simulink model "PosControl_Sim_PID"  (R2018a)
settings: Solver=ode4  StartTime=0.0  StopTime=8  FixedStep=0.001  RelTol=1e-3
InitFcn:
  | Init_control;
values from neighbouring files (symbols this model uses):
  CONSTANTS_ONE_G = 9.8    [Init_control.m]
  DEG2RAD = 0.0174533    [Init_control.m]
  FLT_EPSILON = 1e-5    (= 1e-05)    [Init_control.m]
  MAX_CONTROL_ANGLE_RATE_PITCH = 220    [Init_control.m]
  MAX_CONTROL_ANGLE_RATE_ROLL = 220    [Init_control.m]
  MAX_CONTROL_ANGLE_RATE_Y = 200    [Init_control.m]
  MAX_CONTROL_VELOCITY_XY = 5*2    (= 10)    [Init_control.m]
  MAX_CONTROL_VELOCITY_Z = 3*2    (= 6)    [Init_control.m]
  MC_PITCH_P = 6.5    [Init_control.m]
  MC_PITCHRATE_D = 0.0005    [Init_control.m]
  MC_PITCHRATE_I = 0.2    [Init_control.m]
  MC_PITCHRATE_P = 0.06    [Init_control.m]
  MC_ROLL_P = 11.5    [Init_control.m]
  MC_ROLLRATE_D = 0.0005    [Init_control.m]
  MC_ROLLRATE_I = 0.2    [Init_control.m]
  MC_ROLLRATE_P = 0.055    [Init_control.m]
  MC_YAW_P = 2.8    [Init_control.m]
  MC_YAW_WEIGHT = 0.4    [Init_control.m]
  MC_YAWRATE_D = 0.00    (= 0)    [Init_control.m]
  MC_YAWRATE_I = 0.1    [Init_control.m]
  MC_YAWRATE_P = 0.2    [Init_control.m]
  MPC_THR_MAX = 0.9    [Init_control.m]
  MPC_THR_MIN = 0.06    [Init_control.m]
  MPC_THR_XY_MARG = 0.3    [Init_control.m]
  MPC_TILTMAX_AIR = 90    [Init_control.m]
  MPC_XY_P = 2.2    [Init_control.m]
  MPC_XY_VEL_D_ACC = 0.2    [Init_control.m]
  MPC_XY_VEL_I_ACC = 0.4    [Init_control.m]
  MPC_XY_VEL_P_ACC = 4.0    (= 4)    [Init_control.m]
  MPC_Z_P = 0.8    [Init_control.m]
  MPC_Z_VEL_D_ACC = 0.0    (= 0)    [Init_control.m]
  MPC_Z_VEL_I_ACC = 2.0    (= 2)    [Init_control.m]
  MPC_Z_VEL_P_ACC = 4.0    (= 4)    [Init_control.m]
  Saturation_I_ah = 3.43    [Init_control.m]
  Saturation_I_az = 5    [Init_control.m]
  Saturation_I_RP_Max = 0.3    [Init_control.m]
  Saturation_I_RP_Min = -0.3    [Init_control.m]
  Saturation_I_Y_Max = 0.2    [Init_control.m]
  Saturation_I_Y_Min = -0.2    [Init_control.m]
  THR_HOVER = 0.331    [Init_control.m]
undefined symbols (not defined in the file or in its folder): DiscIntNeverNeededParam, earthRadius, ModelInit_AngEuler, ModelInit_PosE, ModelInit_Rads, ModelInit_RateB, ModelInit_VelB, ModelParam_envGravityAcc, ModelParam_motorCr, ModelParam_motorJm, ModelParam_motorT, ModelParam_motorWb, ModelParam_rotorCm, ModelParam_rotorCt, ModelParam_uavCCm, ModelParam_uavCd, ModelParam_uavJ, ModelParam_uavMass, ModelParam_uavR
libraries: simulink x7, sharedutil x2, aerolibfltsims x2, aerolibanimutils x1
(part 1 of 2)
settings Model: Creator=wsh  LastModifiedBy=truel
settings DebuggingCC: BusObjectLabelMismatch=error
settings CodeAppCC: StateflowObjectComments=on

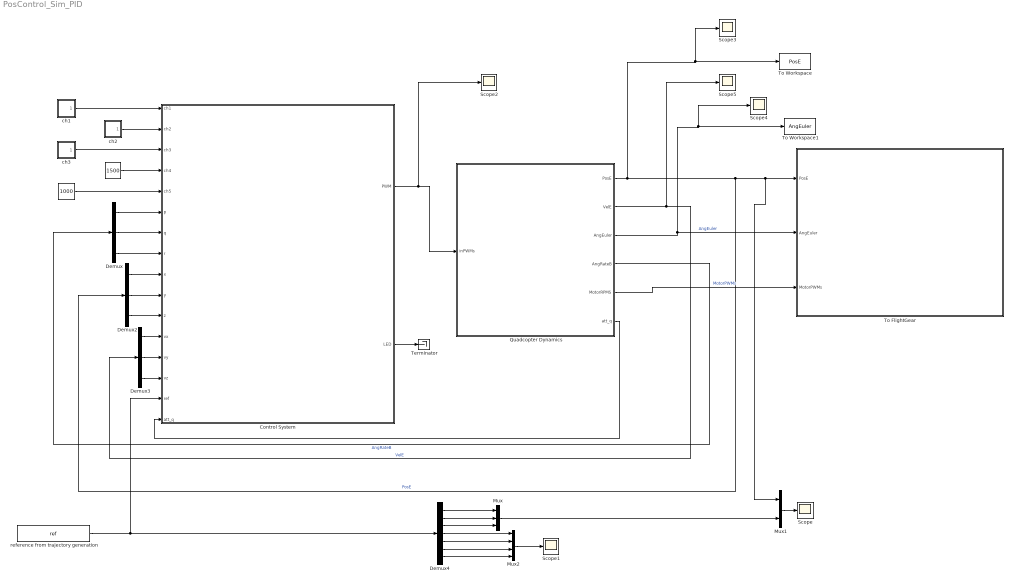
== system PosControl_Sim_PID ==
  " " : Constant  Value=1000  OutDataTypeStr=uint16
  "          " : Constant  Value=1500  OutDataTypeStr=uint16
  Control System : Subsystem
      mask Display: image('icon\pixhawk.png');
  Demux : Demux  Outputs=3
  Demux2 : Demux  Outputs=3
  Demux3 : Demux  Outputs=3
  Demux4 : Demux  Outputs=7
  Mux : Mux  Inputs=3
  Mux1 : Mux  Inputs=2
  Mux2 : Mux
  Quadcopter Dynamics : Subsystem
      mask Display: image('./icon/F450.png');
  Scope{,1..5} (6 alike) : Scope
  Terminator : Terminator
  To FlightGear : Subsystem
      mask Display: image('./icon/FlightGear.png');
  To Workspace : ToWorkspace  VariableName=PosE  SaveFormat=Structure With Time  SampleTime=-1
  To Workspace1 : ToWorkspace  VariableName=AngEuler  SaveFormat=Structure With Time  SampleTime=-1
  ch1 : Subsystem
  ch2 : Subsystem
  ch3 : Subsystem
  reference from trajectory generation : FromWorkspace  VariableName=ref  SampleTime=0
  wires:
  Quadcopter Dynamics/1(PosE) -> Demux2/1, Mux1/1, To FlightGear/1(PosE), To Workspace/1, Scope3/1  "PosE"
  Quadcopter Dynamics/5(MotorRPMS) -> To FlightGear/3(MotorPWMs)  "MotorPWMs"
  Control System/2(LED) -> Terminator/1
  Quadcopter Dynamics/3(AngEuler) -> To Workspace1/1, Scope4/1, To FlightGear/2(AngEuler)  "AngEuler"
  "          "/1 -> Control System/4(ch4)
  Quadcopter Dynamics/4(AngRateB) -> Demux/1  "AngRateB"
  " "/1 -> Control System/5(ch5)
  Demux/1 -> Control System/6(p)
  Demux/2 -> Control System/7(q)
  Demux/3 -> Control System/8(r)
  Demux2/1 -> Control System/9(x)
  Demux2/2 -> Control System/10(y)
  Demux2/3 -> Control System/11(z)
  Demux3/1 -> Control System/12(vx)
  Demux3/2 -> Control System/13(vy)
  Demux3/3 -> Control System/14(vz)
  Quadcopter Dynamics/2(VelE) -> Scope5/1, Demux3/1  "VelE"
  ch2/1(ch2) -> Control System/2(ch2)
  ch3/1(ch3) -> Control System/3(ch3)
  Control System/1(PWM) -> Scope2/1, Quadcopter Dynamics/1(inPWMs)
  reference from trajectory generation/1 -> Control System/15(ref), Demux4/1
  Demux4/1 -> Mux/1
  Demux4/2 -> Mux/2
  Demux4/3 -> Mux/3
  Mux1/1 -> Scope/1
  Mux/1 -> Mux1/2
  Demux4/4 -> Mux2/1
  Demux4/5 -> Mux2/2
  Demux4/6 -> Mux2/3
  Demux4/7 -> Mux2/4
  Mux2/1 -> Scope1/1
  Quadcopter Dynamics/6(att_q) -> Control System/16(att_q)
  ch1/1(ch1) -> Control System/1(ch1)

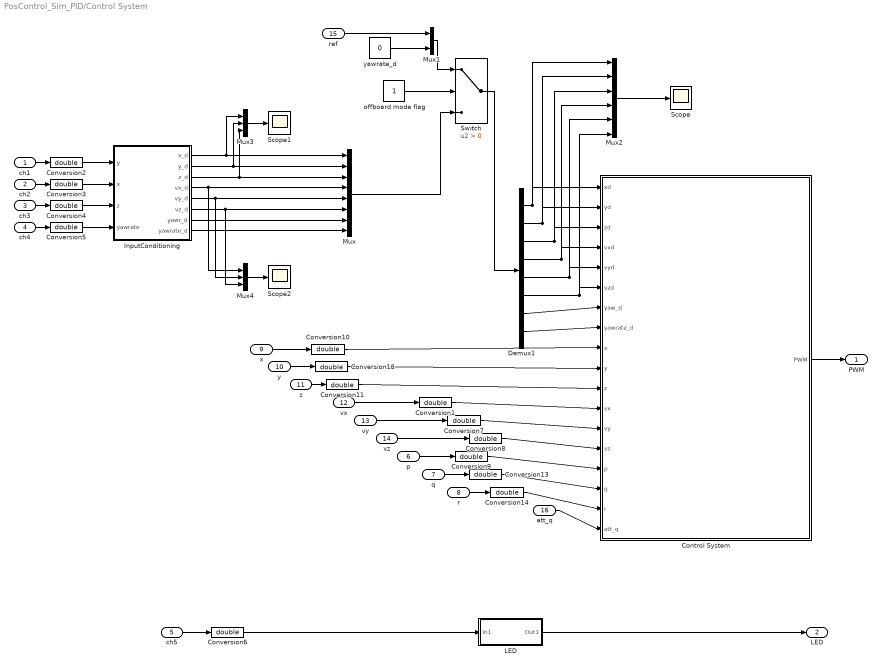
== system PosControl_Sim_PID/Control System ==
  ch1 : Inport  OutDataTypeStr=uint16  PortDimensions=1
  ch2 : Inport  Port=2  OutDataTypeStr=uint16  PortDimensions=1
  ch3 : Inport  Port=3  OutDataTypeStr=uint16  PortDimensions=1
  ch4 : Inport  Port=4  OutDataTypeStr=uint16  PortDimensions=1
  ch5 : Inport  Port=5  OutDataTypeStr=uint16  PortDimensions=1  Interpolate=off
  p : Inport  Port=6  PortDimensions=1
  q : Inport  Port=7  PortDimensions=1
  r : Inport  Port=8  PortDimensions=1
  x : Inport  Port=9
  y : Inport  Port=10
  z : Inport  Port=11
  vx : Inport  Port=12
  vy : Inport  Port=13
  vz : Inport  Port=14
  ref : Inport  Port=15
  att_q : Inport  Port=16  PortDimensions=[1 4]
  Control System : Subsystem
  Conversion{1..11,13..14,18} (14 alike) : DataTypeConversion  OutDataTypeStr=double
  Demux1 : Demux  Outputs=8
  InputConditioning : Subsystem
  "LED " : Subsystem
  Mux : Mux  Inputs=8
  Mux1 : Mux  Inputs=2
  Mux2 : Mux  Inputs=6
  Mux3 : Mux  Inputs=3
  Mux4 : Mux  Inputs=3
  Scope : Scope
  Scope1 : Scope
  Scope2 : Scope
  Switch : Switch  Criteria=u2 > Threshold
  offboard mode flag : Constant
  yawrate_d : Constant  Value=0
  PWM : Outport
  LED : Outport  Port=2  PortDimensions=1
  wires:
  ch3/1 -> Conversion4/1
  ch5/1 -> Conversion6/1
  ch4/1 -> Conversion5/1
  "LED "/1(Out1) -> LED/1
  Conversion6/1 -> "LED "/1(In1)
  Conversion5/1 -> InputConditioning/4("yawrate ")
  Control System/1(PWM) -> PWM/1
  ch1/1 -> Conversion2/1
  ch2/1 -> Conversion3/1
  y/1 -> Conversion18/1
  z/1 -> Conversion11/1
  vy/1 -> Conversion7/1
  Conversion10/1 -> Control System/9(x)
  Conversion18/1 -> Control System/10(y)
  Conversion11/1 -> Control System/11(z)
  Conversion2/1 -> InputConditioning/1(y)
  Conversion3/1 -> InputConditioning/2(x)
  vx/1 -> Conversion1/1
  Conversion1/1 -> Control System/12(vx)
  Conversion7/1 -> Control System/13(vy)
  vz/1 -> Conversion8/1
  Conversion8/1 -> Control System/14(vz)
  p/1 -> Conversion9/1
  q/1 -> Conversion13/1
  r/1 -> Conversion14/1
  Conversion9/1 -> Control System/15(p)
  Conversion13/1 -> Control System/16(q)
  Conversion14/1 -> Control System/17(r)
  Conversion4/1 -> InputConditioning/3(z)
  x/1 -> Conversion10/1
  offboard mode flag/1 -> Switch/2
  ref/1 -> Mux1/1
  yawrate_d/1 -> Mux1/2
  Mux1/1 -> Switch/1
  Mux/1 -> Switch/3
  Switch/1 -> Demux1/1
  Demux1/1 -> Control System/1(xd), Mux2/1
  Demux1/3 -> Control System/3(zd), Mux2/3
  Demux1/4 -> Mux2/4, Control System/4(vxd)
  Demux1/5 -> Mux2/5, Control System/5(vyd)
  Demux1/6 -> Mux2/6, Control System/6(vzd)
  Demux1/8 -> Control System/8(yawrate_d)
  Demux1/7 -> Control System/7(yaw_d)
  att_q/1 -> Control System/18(att_q)
  Mux2/1 -> Scope/1
  Demux1/2 -> Control System/2(yd), Mux2/2
  Mux3/1 -> Scope1/1
  InputConditioning/1(x_d) -> Mux3/1, Mux/1
  InputConditioning/2(y_d) -> Mux3/2, Mux/2
  InputConditioning/3(z_d) -> Mux3/3, Mux/3
  InputConditioning/7(yawr_d) -> Mux/7
  InputConditioning/8(yawrate_d) -> Mux/8
  Mux4/1 -> Scope2/1
  InputConditioning/4(vx_d) -> Mux4/1, Mux/4
  InputConditioning/5(vy_d) -> Mux4/2, Mux/5
  InputConditioning/6(vz_d) -> Mux4/3, Mux/6

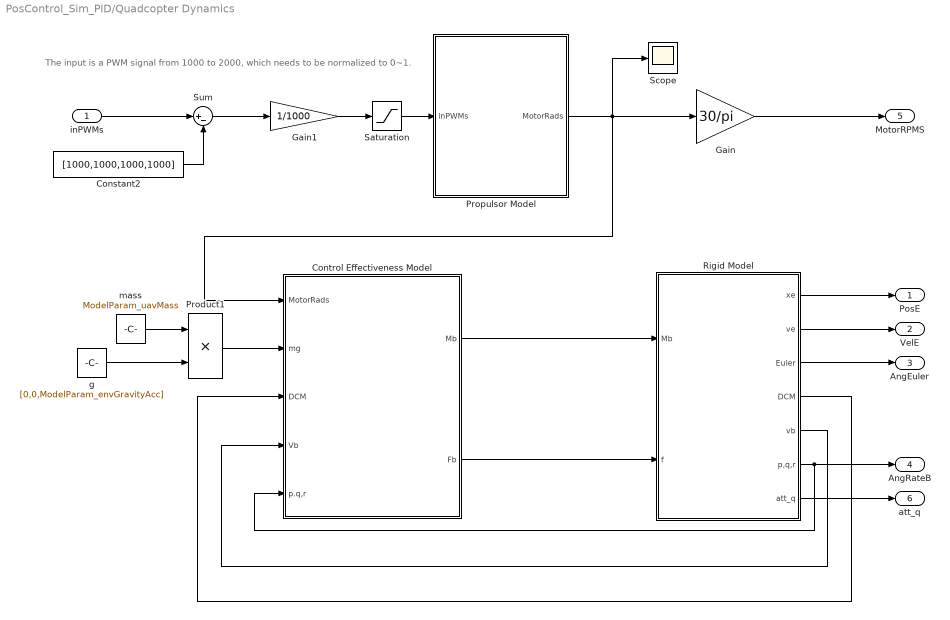
== system PosControl_Sim_PID/Quadcopter Dynamics ==
  note: The input is a PWM signal from 1000 to 2000,
      | which needs to be normalized to 0~1.
  inPWMs : Inport
  Constant2 : Constant  Value=[1000,1000,1000,1000]
  Control Effectiveness Model : Subsystem
  Gain : Gain  Gain=30/pi
  Gain1 : Gain  Gain=1/1000
  Product1 : Product
  Propulsor Model : Subsystem
  Rigid Model : Subsystem
  Saturation : Saturate  UpperLimit=1  LowerLimit=0
  Scope : Scope
  Sum : Sum  Inputs=|+-
  g : Constant  Value=[0,0,ModelParam_envGravityAcc]
  mass : Constant  Value=ModelParam_uavMass
  PosE : Outport
  VelE : Outport  Port=2
  AngEuler : Outport  Port=3
  AngRateB : Outport  Port=4
  MotorRPMS : Outport  Port=5
  att_q : Outport  Port=6
  wires:
  Saturation/1 -> Propulsor Model/1(inPWMs)
  Rigid Model/6("p,q,r ") -> Control Effectiveness Model/5(p.q,r), AngRateB/1
  mass/1 -> Product1/1
  Rigid Model/4(DCM) -> Control Effectiveness Model/3(DCM)
  Propulsor Model/1(MotorRads) -> Scope/1, Gain/1, Control Effectiveness Model/1(MotorRads)
  Gain1/1 -> Saturation/1
  Rigid Model/2(ve) -> VelE/1
  Sum/1 -> Gain1/1
  Product1/1 -> Control Effectiveness Model/2(mg)
  Rigid Model/5("vb ") -> Control Effectiveness Model/4(Vb)
  Rigid Model/1("xe ") -> PosE/1
  Rigid Model/3(Euler) -> AngEuler/1
  Control Effectiveness Model/1(Mb) -> Rigid Model/1(Mb)
  inPWMs/1 -> Sum/1
  Control Effectiveness Model/2(Fb) -> Rigid Model/2(f)
  Constant2/1 -> Sum/2
  g/1 -> Product1/2
  Gain/1 -> MotorRPMS/1
  Rigid Model/7(att_q) -> att_q/1

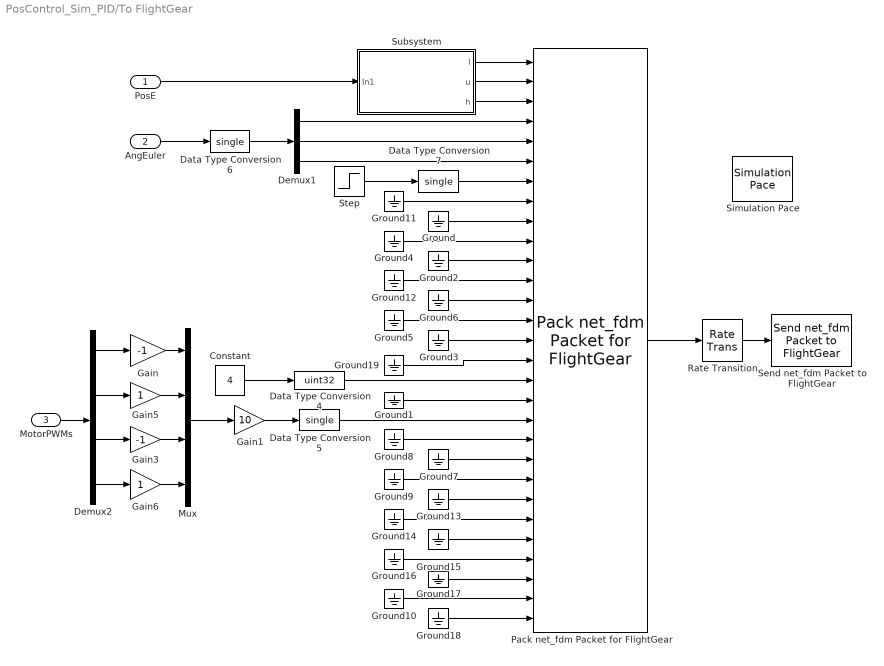
== system PosControl_Sim_PID/To FlightGear ==
  PosE : Inport
  AngEuler : Inport  Port=2
  MotorPWMs : Inport  Port=3
  Constant : Constant  Value=4
  Data Type Conversion4 : DataTypeConversion  OutDataTypeStr=uint32
  Data Type Conversion5 : DataTypeConversion  OutDataTypeStr=single
  Data Type Conversion6 : DataTypeConversion  OutDataTypeStr=single
  Data Type Conversion7 : DataTypeConversion  OutDataTypeStr=single
  Demux1 : Demux  Outputs=3
  Demux2 : Demux
  Gain : Gain  Gain=-1
  Gain1 : Gain  Gain=10
  Gain3 : Gain  Gain=-1
  Gain5 : Gain
  Gain6 : Gain
  Ground{,1..19} (20 alike) : Ground
  Mux : Mux
  Pack net_fdm Packet for FlightGear : aerolibfltsims/Pack net_fdm Packet for FlightGear  FlightGearVersion=v2016.1  ShowPositionAttitudeInputs=on  ShowVelocityAccelerationInputs=off  ShowControlSurfacePositionInputs=on  ShowEngineFuelInputs=on  ShowLandingGearInputs=off  ShowEnvironmentInputs=off  SampleTime=0.01
      settings: SourceProductName=Aerospace Blockset  SourceProductBaseCode=AE
  Rate Transition : RateTransition
  Send net_fdm Packet to FlightGear : aerolibfltsims/Send net_fdm Packet to FlightGear  DestinationIpAddress=127.0.0.1  DestinationPort=5502  LocalIpPort=-1  varLen=off  SampleTime=0.005
      settings: SourceProductName=Aerospace Blockset  SourceProductBaseCode=AE
  Simulation Pace : aerolibanimutils/Simulation Pace  SimulationPace=1  SleepMode=MATLAB Thread  OutputPaceError=off  SampleTime=-1
      settings: AttributesFormatString=%<SimulationPace> sec/sec
  Step : Step  Time=5  SampleTime=0
  Subsystem : Subsystem
  wires:
  Pack net_fdm Packet for FlightGear/1 -> Rate Transition/1
  Data Type Conversion7/1 -> Pack net_fdm Packet for FlightGear/7
  Ground8/1 -> Pack net_fdm Packet for FlightGear/20
  Ground/1 -> Pack net_fdm Packet for FlightGear/9
  Ground7/1 -> Pack net_fdm Packet for FlightGear/21
  Ground9/1 -> Pack net_fdm Packet for FlightGear/22
  Ground13/1 -> Pack net_fdm Packet for FlightGear/23
  Ground14/1 -> Pack net_fdm Packet for FlightGear/24
  Ground15/1 -> Pack net_fdm Packet for FlightGear/25
  Ground16/1 -> Pack net_fdm Packet for FlightGear/26
  Ground17/1 -> Pack net_fdm Packet for FlightGear/27
  Ground10/1 -> Pack net_fdm Packet for FlightGear/28
  Ground18/1 -> Pack net_fdm Packet for FlightGear/29
  Step/1 -> Data Type Conversion7/1
  Data Type Conversion4/1 -> Pack net_fdm Packet for FlightGear/17
  Ground1/1 -> Pack net_fdm Packet for FlightGear/18
  Ground3/1 -> Pack net_fdm Packet for FlightGear/15
  Ground5/1 -> Pack net_fdm Packet for FlightGear/14
  Ground6/1 -> Pack net_fdm Packet for FlightGear/13
  Ground4/1 -> Pack net_fdm Packet for FlightGear/10
  Ground11/1 -> Pack net_fdm Packet for FlightGear/8
  Constant/1 -> Data Type Conversion4/1
  Data Type Conversion5/1 -> Pack net_fdm Packet for FlightGear/19
  Ground2/1 -> Pack net_fdm Packet for FlightGear/11
  Ground12/1 -> Pack net_fdm Packet for FlightGear/12
  AngEuler/1 -> Data Type Conversion6/1
  MotorPWMs/1 -> Demux2/1
  Mux/1 -> Gain1/1
  Demux2/1 -> Gain/1
  Demux2/3 -> Gain3/1
  Gain/1 -> Mux/1
  Gain3/1 -> Mux/3
  Demux2/2 -> Gain5/1
  Gain5/1 -> Mux/2
  Demux2/4 -> Gain6/1
  Gain6/1 -> Mux/4
  Rate Transition/1 -> Send net_fdm Packet to FlightGear/1
  PosE/1 -> Subsystem/1(In1)
  Subsystem/1("l ") -> Pack net_fdm Packet for FlightGear/1
  Subsystem/2(u) -> Pack net_fdm Packet for FlightGear/2
  Subsystem/3(h) -> Pack net_fdm Packet for FlightGear/3
  Ground19/1 -> Pack net_fdm Packet for FlightGear/16
  Demux1/1 -> Pack net_fdm Packet for FlightGear/4
  Demux1/2 -> Pack net_fdm Packet for FlightGear/5
  Demux1/3 -> Pack net_fdm Packet for FlightGear/6
  Data Type Conversion6/1 -> Demux1/1
  Gain1/1 -> Data Type Conversion5/1

== system PosControl_Sim_PID/ch1 ==
  "  " : Constant  Value=1500  OutDataTypeStr=uint16
  Constant : Constant  Value=0
  Constant1 : Constant  Value=0
  Data Type Conversion : DataTypeConversion  OutDataTypeStr=uint16
  Data Type Conversion1 : DataTypeConversion  OutDataTypeStr=uint16
  Delay : Delay  DelayLength=1500
  Delay1 : Delay  DelayLength=3000
  Sum : Sum  Inputs=|+-
  Sum1 : Sum  Inputs=|++
  ch1 : Outport
  wires:
  "  "/1 -> Sum/1
  Constant/1 -> Data Type Conversion/1
  Delay/1 -> Sum/2
  Data Type Conversion/1 -> Delay/1
  Data Type Conversion1/1 -> Delay1/1
  Constant1/1 -> Data Type Conversion1/1
  Delay1/1 -> Sum1/2
  Sum/1 -> Sum1/1
  Sum1/1 -> ch1/1

== system PosControl_Sim_PID/ch2 ==
  "  " : Constant  Value=1500  OutDataTypeStr=uint16
  Constant : Constant  Value=150
  Constant1 : Constant  Value=150
  Data Type Conversion : DataTypeConversion  OutDataTypeStr=uint16
  Data Type Conversion1 : DataTypeConversion  OutDataTypeStr=uint16
  Delay : Delay  DelayLength=5000
  Delay1 : Delay  DelayLength=2000
  Sum : Sum  Inputs=|+-
  Sum1 : Sum  Inputs=|++
  ch2 : Outport
  wires:
  "  "/1 -> Sum/1
  Constant/1 -> Data Type Conversion/1
  Delay/1 -> Sum/2
  Data Type Conversion/1 -> Delay/1
  Data Type Conversion1/1 -> Delay1/1
  Constant1/1 -> Data Type Conversion1/1
  Delay1/1 -> Sum1/2
  Sum/1 -> Sum1/1
  Sum1/1 -> ch2/1

== system PosControl_Sim_PID/ch3 ==
  "  " : Constant  Value=1500  OutDataTypeStr=uint16
  Constant : Constant  Value=0
  Constant1 : Constant  Value=0
  Data Type Conversion : DataTypeConversion  OutDataTypeStr=uint16
  Data Type Conversion1 : DataTypeConversion  OutDataTypeStr=uint16
  Delay : Delay  DelayLength=1500
  Delay1 : Delay  DelayLength=5000
  Sum : Sum  Inputs=|+-
  Sum1 : Sum  Inputs=|++
  ch3 : Outport
  wires:
  "  "/1 -> Sum/1
  Constant/1 -> Data Type Conversion/1
  Delay/1 -> Sum/2
  Data Type Conversion/1 -> Delay/1
  Data Type Conversion1/1 -> Delay1/1
  Constant1/1 -> Data Type Conversion1/1
  Delay1/1 -> Sum1/2
  Sum/1 -> Sum1/1
  Sum1/1 -> ch3/1

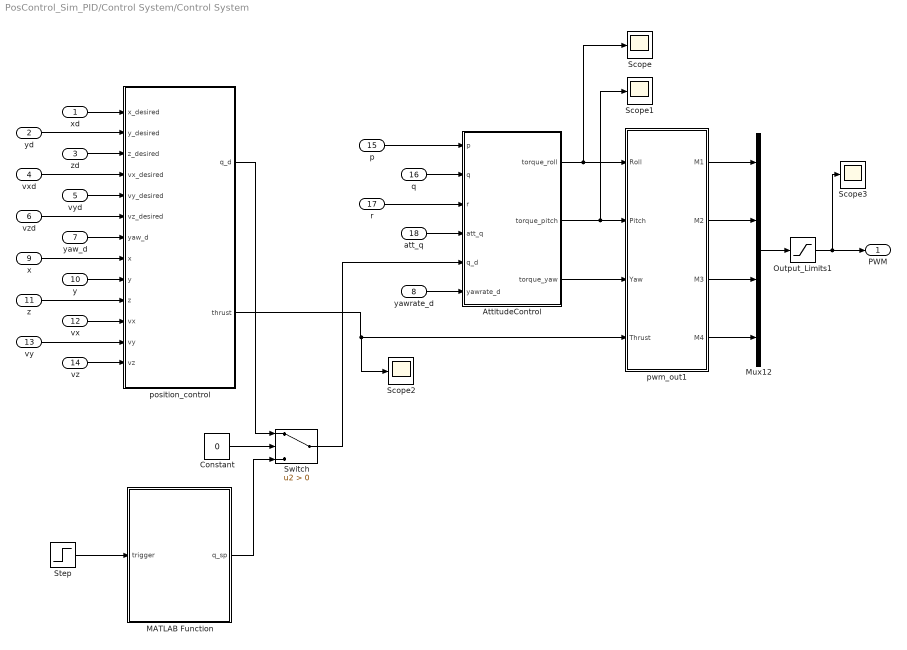
== system PosControl_Sim_PID/Control System/Control System ==
  xd : Inport
  yd : Inport  Port=2
  zd : Inport  Port=3
  vxd : Inport  Port=4
  vyd : Inport  Port=5
  vzd : Inport  Port=6
  yaw_d : Inport  Port=7
  yawrate_d : Inport  Port=8
  x : Inport  Port=9
  y : Inport  Port=10
  z : Inport  Port=11
  vx : Inport  Port=12
  vy : Inport  Port=13
  vz : Inport  Port=14
  p : Inport  Port=15  PortDimensions=1
  q : Inport  Port=16
  r : Inport  Port=17  PortDimensions=1
  att_q : Inport  Port=18
  AttitudeControl : Subsystem
  Constant : Constant  Value=0
  MATLAB Function : MATLAB Function  TreatAsAtomicUnit=on
  Mux12 : Mux
  Output_Limits1 : Saturate  UpperLimit=2000  LowerLimit=1000
  Scope{,1..3} (4 alike) : Scope
  Step : Step  Time=3  SampleTime=0
  Switch : Switch  Criteria=u2 > Threshold
  position_control : Subsystem
  pwm_out1 : MATLAB Function  SystemSampleTime=0.004
  PWM : Outport
  wires:
  q/1 -> AttitudeControl/2(q)
  p/1 -> AttitudeControl/1(p)
  vy/1 -> position_control/12(vy)
  vx/1 -> position_control/11(vx)
  vxd/1 -> position_control/4(vx_desired)
  y/1 -> position_control/9(y)
  vzd/1 -> position_control/6(vz_desired)
  x/1 -> position_control/8(x)
  z/1 -> position_control/10(z)
  vz/1 -> position_control/13(vz)
  xd/1 -> position_control/1(x_desired)
  yd/1 -> position_control/2(y_desired)
  vyd/1 -> position_control/5(vy_desired)
  zd/1 -> position_control/3(z_desired)
  Mux12/1 -> Output_Limits1/1
  pwm_out1/1(M1) -> Mux12/1
  pwm_out1/3(M3) -> Mux12/3
  pwm_out1/2(M2) -> Mux12/2
  pwm_out1/4(M4) -> Mux12/4
  Output_Limits1/1 -> Scope3/1, PWM/1
  AttitudeControl/1(torque_roll) -> Scope/1, pwm_out1/1(Roll)
  AttitudeControl/2(torque_pitch) -> Scope1/1, pwm_out1/2(Pitch)
  AttitudeControl/3(torque_yaw) -> pwm_out1/3(Yaw)
  position_control/2(thrust) -> Scope2/1, pwm_out1/4(Thrust)
  yaw_d/1 -> position_control/7(yaw_d)
  att_q/1 -> AttitudeControl/4(att_q)
  r/1 -> AttitudeControl/3(r)
  yawrate_d/1 -> AttitudeControl/6(yawrate_d)
  Step/1 -> MATLAB Function/1(trigger)
  Constant/1 -> Switch/2
  position_control/1(q_d) -> Switch/1
  MATLAB Function/1(q_sp) -> Switch/3
  Switch/1 -> AttitudeControl/5(q_d)

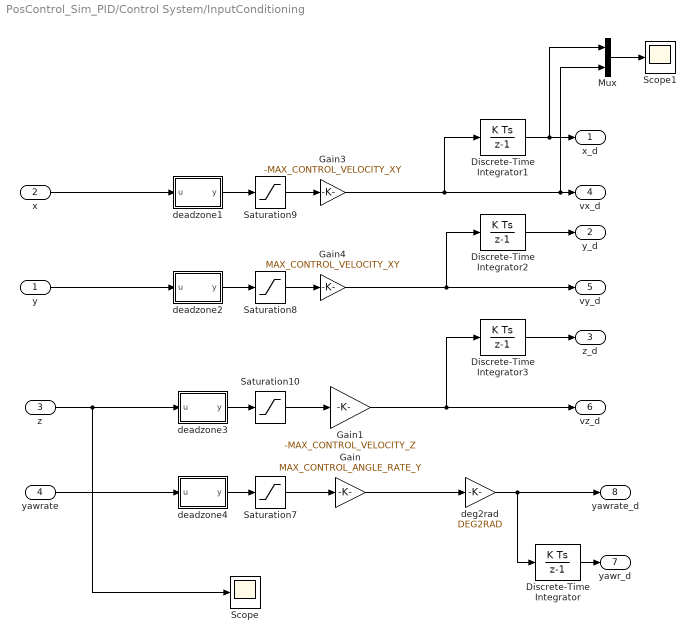
== system PosControl_Sim_PID/Control System/InputConditioning ==
  y : Inport
  x : Inport  Port=2
  z : Inport  Port=3
  "yawrate " : Inport  Port=4
  Discrete-Time Integrator{,1..3} (4 alike) : DiscreteIntegrator  SampleTime=-1  LimitOutput=on  ICPrevOutput=DiscIntNeverNeededParam  ICPrevScaledInput=DiscIntNeverNeededParam
  Gain : Gain  Gain=MAX_CONTROL_ANGLE_RATE_Y
  Gain1 : Gain  Gain=-MAX_CONTROL_VELOCITY_Z  OutDataTypeStr=Inherit: Inherit via back propagation
  Gain3 : Gain  Gain=-MAX_CONTROL_VELOCITY_XY  OutDataTypeStr=Inherit: Inherit via back propagation
  Gain4 : Gain  Gain=MAX_CONTROL_VELOCITY_XY  OutDataTypeStr=Inherit: Inherit via back propagation
  Mux : Mux  Inputs=2
  Saturation{7..10} (4 alike) : Saturate  UpperLimit=1  LowerLimit=-1
  Scope : Scope
  Scope1 : Scope
  deadzone1 : MATLAB Function  TreatAsAtomicUnit=on
  deadzone2 : MATLAB Function  TreatAsAtomicUnit=on
  deadzone3 : MATLAB Function  TreatAsAtomicUnit=on
  deadzone4 : MATLAB Function  TreatAsAtomicUnit=on
  deg2rad : Gain  Gain=DEG2RAD
  x_d : Outport
  y_d : Outport  Port=2
  z_d : Outport  Port=3
  vx_d : Outport  Port=4
  vy_d : Outport  Port=5
  vz_d : Outport  Port=6
  yawr_d : Outport  Port=7
  yawrate_d : Outport  Port=8
  wires:
  Saturation10/1 -> Gain1/1
  Saturation7/1 -> Gain/1
  deadzone3/1(y) -> Saturation10/1
  deadzone4/1(y) -> Saturation7/1
  Gain/1 -> deg2rad/1
  z/1 -> Scope/1, deadzone3/1(u)
  "yawrate "/1 -> deadzone4/1(u)
  deadzone1/1(y) -> Saturation9/1
  Saturation9/1 -> Gain3/1
  x/1 -> deadzone1/1(u)
  Saturation8/1 -> Gain4/1
  deadzone2/1(y) -> Saturation8/1
  y/1 -> deadzone2/1(u)
  Gain4/1 -> Discrete-Time Integrator2/1, vy_d/1
  deg2rad/1 -> Discrete-Time Integrator/1, yawrate_d/1
  Discrete-Time Integrator/1 -> yawr_d/1
  Gain3/1 -> Discrete-Time Integrator1/1, Mux/2, vx_d/1
  Discrete-Time Integrator1/1 -> Mux/1, x_d/1
  Discrete-Time Integrator2/1 -> y_d/1
  Discrete-Time Integrator3/1 -> z_d/1
  Gain1/1 -> Discrete-Time Integrator3/1, vz_d/1
  Mux/1 -> Scope1/1

== system PosControl_Sim_PID/Control System/LED  ==
  In1 : Inport
  Compare To Constant3 : simulink/Logic and Bit Operations/Compare To Constant  relop=>=  const=uint16(1500)  OutDataTypeStr=boolean
  Out1 : Outport
  wires:
  Compare To Constant3/1 -> Out1/1
  In1/1 -> Compare To Constant3/1

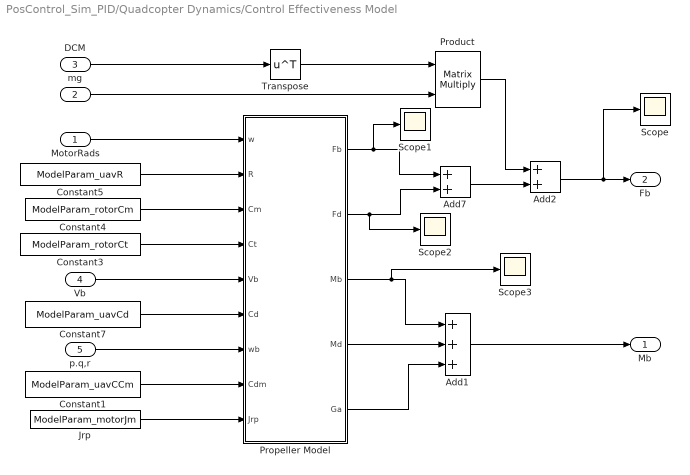
== system PosControl_Sim_PID/Quadcopter Dynamics/Control Effectiveness Model ==
  MotorRads : Inport
  mg : Inport  Port=2
  DCM : Inport  Port=3
  Vb : Inport  Port=4
  p.q,r : Inport  Port=5
  Add1 : Sum  Inputs=+++
  Add2 : Sum
  Add7 : Sum
  Constant1 : Constant  Value=ModelParam_uavCCm
  Constant3 : Constant  Value=ModelParam_rotorCt
  Constant4 : Constant  Value=ModelParam_rotorCm
  Constant5 : Constant  Value=ModelParam_uavR
  Constant7 : Constant  Value=ModelParam_uavCd
  Jrp : Constant  Value=ModelParam_motorJm
  Product : Product  Multiplication=Matrix(*)
  Propeller Model : MATLAB Function  TreatAsAtomicUnit=on
  Scope{,1..3} (4 alike) : Scope
  Transpose : Math  Operator=transpose  SaturateOnIntegerOverflow=on
  Mb : Outport
  Fb : Outport  Port=2
  wires:
  Add2/1 -> Scope/1, Fb/1
  Constant3/1 -> Propeller Model/4(Ct)
  Propeller Model/2(Fd) -> Scope2/1, Add7/2
  Add7/1 -> Add2/2
  Propeller Model/1(Fb) -> Scope1/1, Add7/1
  Product/1 -> Add2/1
  mg/1 -> Product/2
  DCM/1 -> Transpose/1
  Constant7/1 -> Propeller Model/6(Cd)
  Vb/1 -> Propeller Model/5(Vb)
  Constant5/1 -> Propeller Model/2(R)
  Constant4/1 -> Propeller Model/3(Cm)
  MotorRads/1 -> Propeller Model/1(w)
  Transpose/1 -> Product/1
  Propeller Model/3(Mb) -> Scope3/1, Add1/1
  Propeller Model/4(Md) -> Add1/2
  Add1/1 -> Mb/1
  p.q,r/1 -> Propeller Model/7(wb)
  Constant1/1 -> Propeller Model/8(Cdm)
  Jrp/1 -> Propeller Model/9(Jrp)
  Propeller Model/5(Ga) -> Add1/3

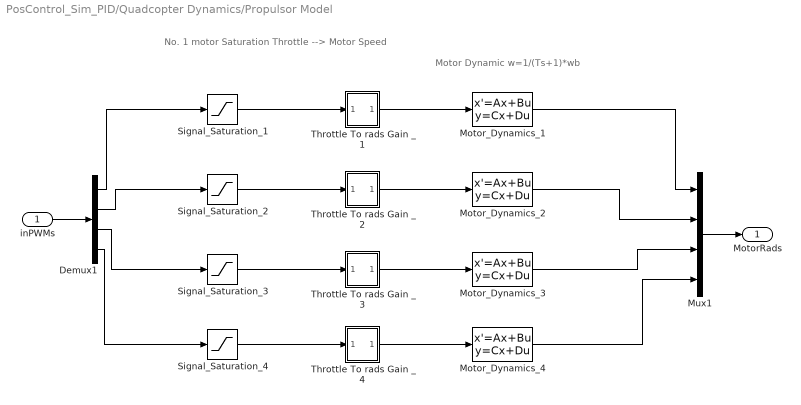
== system PosControl_Sim_PID/Quadcopter Dynamics/Propulsor Model ==
  note: Motor Dynamic
      | w=1/(Ts+1)*wb
  note: No. 1 motor
      |
      |          Saturation             Throttle --> Motor Speed
  inPWMs : Inport
  Demux1 : Demux
  Motor_Dynamics_{1..4} (4 alike) : StateSpace  A=-1/ModelParam_motorT  C=1/ModelParam_motorT  D=0  InitialCondition=ModelInit_Rads*ModelParam_motorT
  Mux1 : Mux
  Signal_Saturation_{1..4} (4 alike) : Saturate  UpperLimit=1  LowerLimit=0
  Throttle To rads Gain _1 : Subsystem
  Throttle To rads Gain _2 : Subsystem
  Throttle To rads Gain _3 : Subsystem
  Throttle To rads Gain _4 : Subsystem
  MotorRads : Outport
  wires:
  Throttle To rads Gain _4/1(Out5) -> Motor_Dynamics_4/1
  Signal_Saturation_4/1 -> Throttle To rads Gain _4/1(In5)
  Signal_Saturation_3/1 -> Throttle To rads Gain _3/1(In5)
  Signal_Saturation_2/1 -> Throttle To rads Gain _2/1(In5)
  Motor_Dynamics_4/1 -> Mux1/4
  Motor_Dynamics_3/1 -> Mux1/3
  Motor_Dynamics_2/1 -> Mux1/2
  Motor_Dynamics_1/1 -> Mux1/1
  Signal_Saturation_1/1 -> Throttle To rads Gain _1/1(In5)
  Mux1/1 -> MotorRads/1
  Throttle To rads Gain _3/1(Out5) -> Motor_Dynamics_3/1
  Throttle To rads Gain _2/1(Out5) -> Motor_Dynamics_2/1
  Throttle To rads Gain _1/1(Out5) -> Motor_Dynamics_1/1
  inPWMs/1 -> Demux1/1
  Demux1/4 -> Signal_Saturation_4/1
  Demux1/3 -> Signal_Saturation_3/1
  Demux1/2 -> Signal_Saturation_2/1
  Demux1/1 -> Signal_Saturation_1/1

== system PosControl_Sim_PID/Quadcopter Dynamics/Rigid Model ==
  Mb : Inport
  f : Inport  Port=2
  Rigid-Body Dynamic Model : Subsystem
  "Rigid-Body Kinematic Model " : Subsystem
  "xe " : Outport
  ve : Outport  Port=2
  Euler : Outport  Port=3
  DCM : Outport  Port=4
  "vb " : Outport  Port=5
  "p,q,r " : Outport  Port=6
  att_q : Outport  Port=7
  wires:
  Rigid-Body Dynamic Model/1("p,q,r ") -> "Rigid-Body Kinematic Model "/1(pqr), "p,q,r "/1
  "Rigid-Body Kinematic Model "/1(Euler) -> Euler/1
  "Rigid-Body Kinematic Model "/3(DCM) -> Rigid-Body Dynamic Model/3(DCM), DCM/1
  Mb/1 -> Rigid-Body Dynamic Model/1(Mb)
  f/1 -> Rigid-Body Dynamic Model/2(f)
  Rigid-Body Dynamic Model/2(ve) -> "Rigid-Body Kinematic Model "/2(ve), ve/1
  Rigid-Body Dynamic Model/3("vb ") -> "vb "/1
  "Rigid-Body Kinematic Model "/2("xe ") -> "xe "/1
  "Rigid-Body Kinematic Model "/4(att_q) -> att_q/1

== system PosControl_Sim_PID/To FlightGear/Subsystem ==
  In1 : Inport
  Constant1 : Constant  Value=5  VectorParams1D=off
  Constant2 : Constant  Value=-2.1361  VectorParams1D=off
  Constant3 : Constant  Value=0.65673  VectorParams1D=off
  Demux : Demux  Outputs=3
  Gain1 : Gain  Gain=10/earthRadius
  Gain2 : Gain  Gain=10/earthRadius
  Gain4 : Gain
  Gain8 : Gain  Gain=-10
  Sum10 : Sum  Inputs=|++
  Sum8 : Sum  Inputs=|++
  Sum9 : Sum  Inputs=|++
  "l " : Outport
  u : Outport  Port=2
  h : Outport  Port=3
  wires:
  Constant3/1 -> Sum9/2
  Constant1/1 -> Sum10/2
  Demux/1 -> Gain4/1
  Demux/3 -> Gain8/1
  Constant2/1 -> Sum8/2
  Gain2/1 -> Sum9/1
  Gain1/1 -> Sum8/1
  Gain8/1 -> Sum10/1
  Demux/2 -> Gain1/1
  Gain4/1 -> Gain2/1
  Sum10/1 -> h/1
  Sum9/1 -> u/1
  In1/1 -> Demux/1
  Sum8/1 -> "l "/1

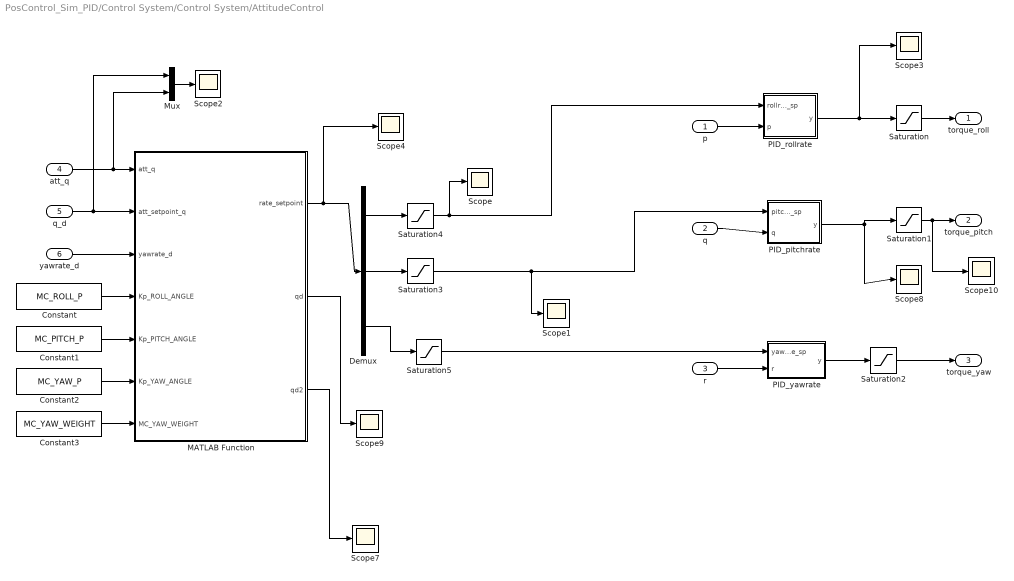
== system PosControl_Sim_PID/Control System/Control System/AttitudeControl ==
  p : Inport
  q : Inport  Port=2
  r : Inport  Port=3
  att_q : Inport  Port=4
  q_d : Inport  Port=5
  yawrate_d : Inport  Port=6
  Constant : Constant  Value=MC_ROLL_P
  Constant1 : Constant  Value=MC_PITCH_P
  Constant2 : Constant  Value=MC_YAW_P
  Constant3 : Constant  Value=MC_YAW_WEIGHT
  Demux : Demux  Outputs=3
  MATLAB Function : MATLAB Function  TreatAsAtomicUnit=on
  Mux : Mux  Inputs=2
  PID_pitchrate : Subsystem
  PID_rollrate : Subsystem
  PID_yawrate : Subsystem
  Saturation : Saturate  UpperLimit=1  LowerLimit=-1
  Saturation1 : Saturate  UpperLimit=1  LowerLimit=-1
  Saturation2 : Saturate
  Saturation3 : Saturate  UpperLimit=MAX_CONTROL_ANGLE_RATE_PITCH  LowerLimit=-MAX_CONTROL_ANGLE_RATE_PITCH
  Saturation4 : Saturate  UpperLimit=MAX_CONTROL_ANGLE_RATE_ROLL  LowerLimit=-MAX_CONTROL_ANGLE_RATE_ROLL
  Saturation5 : Saturate  UpperLimit=MAX_CONTROL_ANGLE_RATE_PITCH  LowerLimit=-MAX_CONTROL_ANGLE_RATE_PITCH
  Scope{,1..4,7..10} (9 alike) : Scope
  torque_roll : Outport
  torque_pitch : Outport  Port=2
  torque_yaw : Outport  Port=3
  wires:
  PID_pitchrate/1(y) -> Saturation1/1, Scope8/1
  PID_yawrate/1(y) -> Saturation2/1
  Saturation/1 -> torque_roll/1
  Saturation1/1 -> torque_pitch/1, Scope10/1
  Saturation2/1 -> torque_yaw/1
  att_q/1 -> Mux/2, MATLAB Function/1(att_q)
  q_d/1 -> Mux/1, MATLAB Function/2(att_setpoint_q)
  MATLAB Function/1(rate_setpoint) -> Demux/1, Scope4/1
  Demux/1 -> Saturation4/1
  Demux/2 -> Saturation3/1
  Demux/3 -> Saturation5/1
  Saturation4/1 -> PID_rollrate/1(rollrate_sp), Scope/1
  Saturation3/1 -> PID_pitchrate/1(pitchrate_sp), Scope1/1
  yawrate_d/1 -> MATLAB Function/3(yawrate_d)
  Constant/1 -> MATLAB Function/4(Kp_ROLL_ANGLE)
  Constant3/1 -> MATLAB Function/7(MC_YAW_WEIGHT)
  Constant2/1 -> MATLAB Function/6(Kp_YAW_ANGLE)
  Constant1/1 -> MATLAB Function/5(Kp_PITCH_ANGLE)
  Mux/1 -> Scope2/1
  PID_rollrate/1(y) -> Scope3/1, Saturation/1
  MATLAB Function/3(qd2) -> Scope7/1
  MATLAB Function/2(qd) -> Scope9/1
  p/1 -> PID_rollrate/2(p)
  q/1 -> PID_pitchrate/2(q)
  Saturation5/1 -> PID_yawrate/1(yawrare_sp)
  r/1 -> PID_yawrate/2(r)

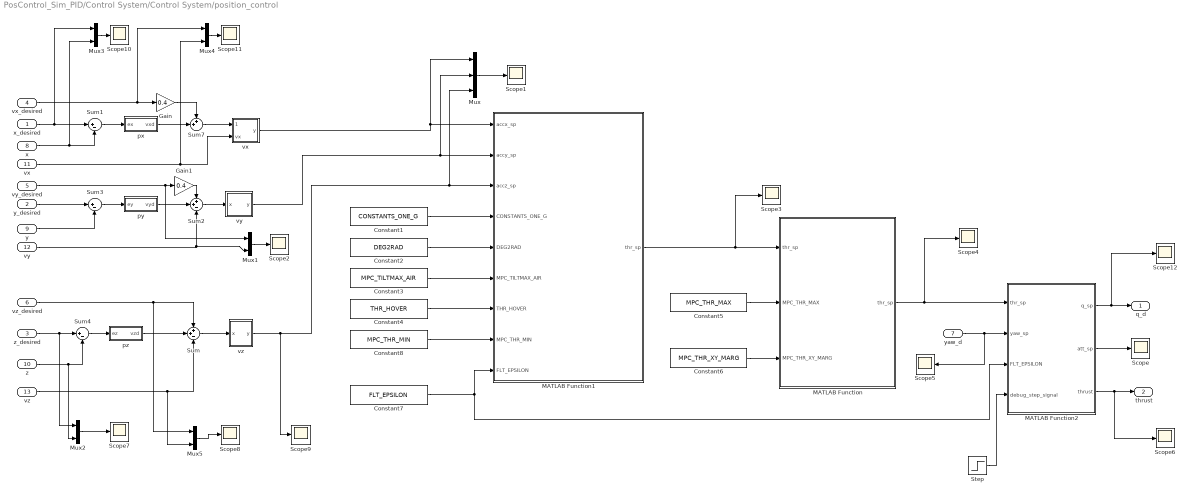
== system PosControl_Sim_PID/Control System/Control System/position_control ==
  x_desired : Inport
  y_desired : Inport  Port=2
  z_desired : Inport  Port=3
  vx_desired : Inport  Port=4
  vy_desired : Inport  Port=5
  vz_desired : Inport  Port=6
  yaw_d : Inport  Port=7
  x : Inport  Port=8
  y : Inport  Port=9
  z : Inport  Port=10
  vx : Inport  Port=11
  vy : Inport  Port=12
  vz : Inport  Port=13
  Constant1 : Constant  Value=CONSTANTS_ONE_G
  Constant2 : Constant  Value=DEG2RAD
  Constant3 : Constant  Value=MPC_TILTMAX_AIR
  Constant4 : Constant  Value=THR_HOVER
  Constant5 : Constant  Value=MPC_THR_MAX
  Constant6 : Constant  Value=MPC_THR_XY_MARG
  Constant7 : Constant  Value=FLT_EPSILON
  Constant8 : Constant  Value=MPC_THR_MIN
  Gain : Gain  Gain=0.4
  Gain1 : Gain  Gain=0.4
  MATLAB Function : MATLAB Function  TreatAsAtomicUnit=on
  MATLAB Function1 : MATLAB Function  TreatAsAtomicUnit=on
  MATLAB Function2 : MATLAB Function  TreatAsAtomicUnit=on
  Mux : Mux  Inputs=3
  Mux{1..5} (5 alike) : Mux  Inputs=2
  Scope{,1..12} (13 alike) : Scope
  Step : Step  Time=3  SampleTime=0
  Sum : Sum  Inputs=++-
  Sum1 : Sum  Inputs=|+-
  Sum2 : Sum  Inputs=++-
  Sum3 : Sum  Inputs=|+-
  Sum4 : Sum  Inputs=|+-
  Sum7 : Sum  Inputs=++|
  px : Subsystem
  py : Subsystem
  pz : Subsystem
  "vx " : Subsystem
  "vy " : Subsystem
  "vz " : Subsystem
  q_d : Outport  PortDimensions=[1, 4]
  thrust : Outport  Port=2
  wires:
  Sum4/1 -> pz/1(ez)
  z/1 -> Mux2/2, Sum4/2
  Sum/1 -> "vz "/1(x)
  vz/1 -> Mux5/2, Sum/3
  x/1 -> Mux3/2, Sum1/2
  y/1 -> Sum3/2
  Sum3/1 -> py/1(ey)
  y_desired/1 -> Sum3/1
  vy/1 -> Mux1/2, Sum2/3
  Sum2/1 -> "vy "/1(x)
  Sum7/1 -> "vx "/1(vx_d)
  Sum1/1 -> px/1(ex)
  vy_desired/1 -> Gain1/1, Mux1/1
  z_desired/1 -> Mux2/1, Sum4/1
  vz_desired/1 -> Mux5/1, Sum/1
  py/1(vyd) -> Sum2/2
  vx_desired/1 -> Gain/1, Mux4/1
  x_desired/1 -> Mux3/1, Sum1/1
  yaw_d/1 -> Scope5/1, MATLAB Function2/2(yaw_sp)
  "vx "/1(y) -> Mux/1, MATLAB Function1/1(accx_sp)
  "vy "/1(y) -> Mux/2, MATLAB Function1/2(accy_sp)
  MATLAB Function2/1(q_sp) -> Scope12/1, q_d/1
  MATLAB Function2/2(att_sp) -> Scope/1
  MATLAB Function2/3(thrust) -> Scope6/1, thrust/1
  Constant1/1 -> MATLAB Function1/4(CONSTANTS_ONE_G)
  Constant2/1 -> MATLAB Function1/5(DEG2RAD)
  Constant3/1 -> MATLAB Function1/6(MPC_TILTMAX_AIR)
  Constant4/1 -> MATLAB Function1/7(THR_HOVER)
  Constant5/1 -> MATLAB Function/2(MPC_THR_MAX)
  MATLAB Function1/1(thr_sp) -> Scope3/1, MATLAB Function/1("thr_sp ")
  MATLAB Function/1(thr_sp) -> Scope4/1, MATLAB Function2/1(thr_sp)
  Constant6/1 -> MATLAB Function/3(MPC_THR_XY_MARG)
  Constant7/1 -> MATLAB Function1/9(FLT_EPSILON), MATLAB Function2/3(FLT_EPSILON)
  Constant8/1 -> MATLAB Function1/8(MPC_THR_MIN)
  Mux/1 -> Scope1/1
  Mux1/1 -> Scope2/1
  Mux2/1 -> Scope7/1
  "vz "/1(y) -> Scope9/1, Mux/3, MATLAB Function1/3(accz_sp)
  Mux3/1 -> Scope10/1
  vx/1 -> "vx "/2(vx), Mux4/2
  Mux4/1 -> Scope11/1
  Mux5/1 -> Scope8/1
  pz/1(vzd) -> Sum/2
  Step/1 -> MATLAB Function2/4(debug_step_signal)
  px/1(vxd) -> Sum7/2
  Gain/1 -> Sum7/1
  Gain1/1 -> Sum2/1

== system PosControl_Sim_PID/Quadcopter Dynamics/Propulsor Model/Throttle To rads Gain _1 ==
  In5 : Inport
  Constant : Constant  Value=ModelParam_motorWb
  Gain : Gain  Gain=ModelParam_motorCr
  Sum1 : Sum  Inputs=++|
  Out5 : Outport
  wires:
  Constant/1 -> Sum1/1
  Gain/1 -> Sum1/2
  In5/1 -> Gain/1
  Sum1/1 -> Out5/1

== system PosControl_Sim_PID/Quadcopter Dynamics/Propulsor Model/Throttle To rads Gain _2 ==
  In5 : Inport
  Constant : Constant  Value=ModelParam_motorWb
  Gain : Gain  Gain=ModelParam_motorCr
  Sum1 : Sum  Inputs=++|
  Out5 : Outport
  wires:
  Sum1/1 -> Out5/1
  In5/1 -> Gain/1
  Gain/1 -> Sum1/2
  Constant/1 -> Sum1/1

== system PosControl_Sim_PID/Quadcopter Dynamics/Propulsor Model/Throttle To rads Gain _3 ==
  In5 : Inport
  Constant : Constant  Value=ModelParam_motorWb
  Gain : Gain  Gain=ModelParam_motorCr
  Sum1 : Sum  Inputs=++|
  Out5 : Outport
  wires:
  Constant/1 -> Sum1/1
  Gain/1 -> Sum1/2
  In5/1 -> Gain/1
  Sum1/1 -> Out5/1

== system PosControl_Sim_PID/Quadcopter Dynamics/Propulsor Model/Throttle To rads Gain _4 ==
  In5 : Inport
  Constant : Constant  Value=ModelParam_motorWb
  Gain : Gain  Gain=ModelParam_motorCr
  Sum1 : Sum  Inputs=++|
  Out5 : Outport
  wires:
  Sum1/1 -> Out5/1
  In5/1 -> Gain/1
  Gain/1 -> Sum1/2
  Constant/1 -> Sum1/1

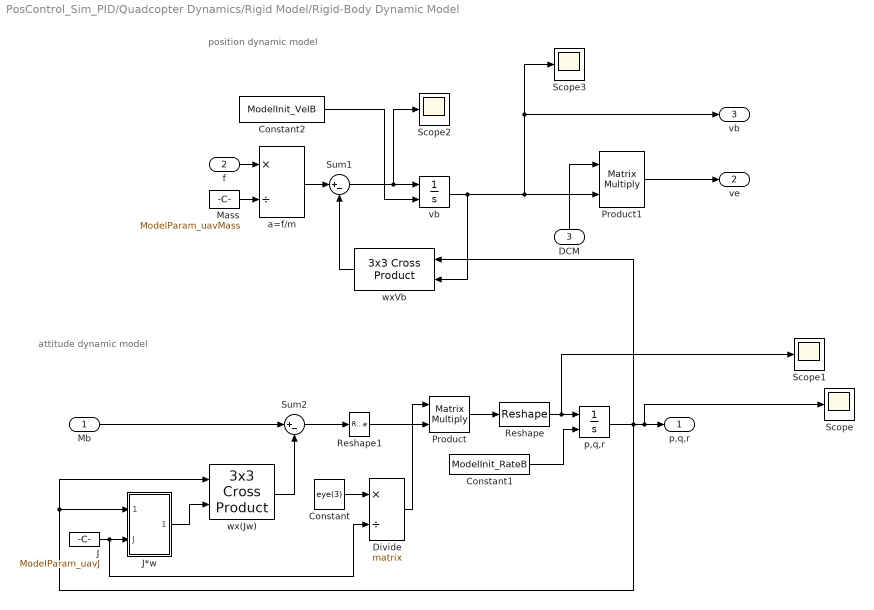
== system PosControl_Sim_PID/Quadcopter Dynamics/Rigid Model/Rigid-Body Dynamic Model ==
  note: attitude dynamic model
  note: position dynamic model
  Mb : Inport
  f : Inport  Port=2
  DCM : Inport  Port=3
  " Mass " : Constant  Value=ModelParam_uavMass
  Constant : Constant  Value=eye(3)
  Constant1 : Constant  Value=ModelInit_RateB
  Constant2 : Constant  Value=ModelInit_VelB
  Divide : Product  Inputs=*/  Multiplication=Matrix(*)
  "J " : Constant  Value=ModelParam_uavJ
  J*w : Subsystem
  Product : Product  Multiplication=Matrix(*)
  Product1 : Product  Multiplication=Matrix(*)
  Reshape : Reshape  OutputDimensionality=Customize  OutputDimensions=[3,1]
  Reshape1 : Reshape  OutputDimensionality=Column vector (2-D)
  Scope{,1..3} (4 alike) : Scope
  Sum1 : Sum  Inputs=|+-
  Sum2 : Sum  Inputs=|+-
  a=f/m : Product  Inputs=*/
  p,q,r : Integrator  InitialConditionSource=external
  vb : Integrator  InitialConditionSource=external
  wx(Jw) : sharedutil/3x3 Cross Product  aMode=aMode
      settings: SourceProductBaseCode=AE
  wxVb : sharedutil/3x3 Cross Product  aMode=aMode
      settings: SourceProductBaseCode=AE
  "p,q,r " : Outport
  ve : Outport  Port=2
  "vb " : Outport  Port=3
  wires:
  Product/1 -> Reshape/1
  Reshape1/1 -> Product/2
  Constant/1 -> Divide/1
  Divide/1 -> Product/1
  Sum2/1 -> Reshape1/1
  "J "/1 -> Divide/2, J*w/2(J)
  p,q,r/1 -> Scope/1, "p,q,r "/1, J*w/1(p q r), wx(Jw)/1, wxVb/1
  J*w/1("J*w ") -> wx(Jw)/2
  Mb/1 -> Sum2/1
  wx(Jw)/1 -> Sum2/2
  Constant2/1 -> vb/2
  f/1 -> a=f/m/1
  Product1/1 -> ve/1
  wxVb/1 -> Sum1/2
  a=f/m/1 -> Sum1/1
  Sum1/1 -> Scope2/1, vb/1
  vb/1 -> Product1/2, Scope3/1, "vb "/1, wxVb/2
  " Mass "/1 -> a=f/m/2
  DCM/1 -> Product1/1
  Reshape/1 -> Scope1/1, p,q,r/1
  Constant1/1 -> p,q,r/2

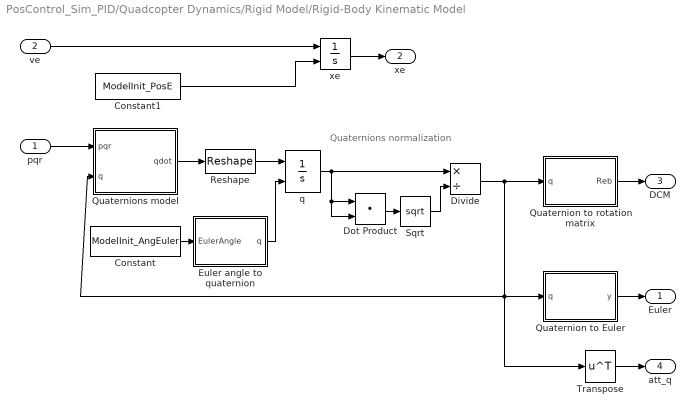
== system PosControl_Sim_PID/Quadcopter Dynamics/Rigid Model/Rigid-Body Kinematic Model  ==
  note: Quaternions
      | normalization
  pqr : Inport
  ve : Inport  Port=2
  Constant : Constant  Value=ModelInit_AngEuler
  Constant1 : Constant  Value=ModelInit_PosE
  Divide : Product  Inputs=*/
  Dot Product : DotProduct  InputSameDT=on  OutDataTypeStr=Inherit: Inherit via internal rule
  Euler angle to quaternion : MATLAB Function
  Quaternion to Euler : MATLAB Function
  Quaternion to rotation matrix : MATLAB Function
  Quaternions model : MATLAB Function  TreatAsAtomicUnit=on
  Reshape : Reshape  OutputDimensionality=Customize  OutputDimensions=[4,1]
  Sqrt : Sqrt  SaturateOnIntegerOverflow=on
  Transpose : Math  Operator=transpose  SaturateOnIntegerOverflow=on
  q : Integrator  InitialConditionSource=external
  xe : Integrator  InitialConditionSource=external
  Euler : Outport
  "xe " : Outport  Port=2
  DCM : Outport  Port=3
  att_q : Outport  Port=4  PortDimensions=[1 4]
  wires:
  Divide/1 -> Quaternion to rotation matrix/1(q), Transpose/1, Quaternions model/2(q), Quaternion to Euler/1(q)
  Dot Product/1 -> Sqrt/1
  pqr/1 -> Quaternions model/1(pqr)
  q/1 -> Divide/1, Dot Product/1, Dot Product/2
  Quaternions model/1(qdot) -> Reshape/1
  Quaternion to rotation matrix/1(Reb) -> DCM/1
  Quaternion to Euler/1(y) -> Euler/1
  Constant/1 -> Euler angle to quaternion/1(EulerAngle)
  Euler angle to quaternion/1(q) -> q/2
  Reshape/1 -> q/1
  ve/1 -> xe/1
  xe/1 -> "xe "/1
  Constant1/1 -> xe/2
  Sqrt/1 -> Divide/2
  Transpose/1 -> att_q/1

== system PosControl_Sim_PID/Control System/Control System/AttitudeControl/PID_pitchrate ==
  pitchrate_sp : Inport
  q : Inport  Port=2
  Derivative Gain : Gain  DisableCoverage=on  Gain=MC_PITCHRATE_D  ParamMin=-100  ParamMax=100  OutMin=-100  OutMax=100
  Discrete Derivative : simulink/Discrete/Discrete Derivative  gainval=1.0  ICPrevScaledInput=0.0  OutMin=[]  OutMax=[]  OutDataType=fixdt(1, 16)  OutScaling=2^-10  DoSatur=off
  Discrete-Time Integrator : DiscreteIntegrator  SampleTime=-1  LimitOutput=on  UpperSaturationLimit=Saturation_I_RP_Max  LowerSaturationLimit=Saturation_I_RP_Min  ICPrevOutput=DiscIntNeverNeededParam  ICPrevScaledInput=DiscIntNeverNeededParam
  Gain : Gain  Gain=MC_PITCHRATE_P
  Gain1 : Gain  Gain=-1
  Integral Gain : Gain  DisableCoverage=on  Gain=MC_PITCHRATE_I
  Scope : Scope
  Scope1 : Scope
  Scope2 : Scope
  Sum : Sum  Inputs=+++
  Sum1 : Sum  Inputs=|+-
  y : Outport  InitialOutput=0
  wires:
  Discrete-Time Integrator/1 -> Scope2/1, Sum/2
  Discrete Derivative/1 -> Scope1/1, Sum/3
  Sum/1 -> y/1
  Gain/1 -> Scope/1, Sum/1
  Derivative Gain/1 -> Discrete Derivative/1
  Integral Gain/1 -> Discrete-Time Integrator/1
  pitchrate_sp/1 -> Sum1/1
  q/1 -> Gain1/1, Sum1/2
  Sum1/1 -> Gain/1, Integral Gain/1
  Gain1/1 -> Derivative Gain/1

== system PosControl_Sim_PID/Control System/Control System/AttitudeControl/PID_rollrate ==
  rollrate_sp : Inport
  p : Inport  Port=2
  Derivative Gain : Gain  DisableCoverage=on  Gain=MC_ROLLRATE_D  ParamMin=-100  ParamMax=100  OutMin=-100  OutMax=100
  Discrete Derivative : simulink/Discrete/Discrete Derivative  gainval=1.0  ICPrevScaledInput=0.0  OutMin=[]  OutMax=[]  OutDataType=fixdt(1, 16)  OutScaling=2^-10  DoSatur=off
  Discrete-Time Integrator : DiscreteIntegrator  SampleTime=-1  LimitOutput=on  UpperSaturationLimit=Saturation_I_RP_Max  LowerSaturationLimit=Saturation_I_RP_Min  ICPrevOutput=DiscIntNeverNeededParam  ICPrevScaledInput=DiscIntNeverNeededParam
  Gain : Gain  Gain=MC_ROLLRATE_P
  Gain1 : Gain  Gain=-1
  Integral Gain : Gain  DisableCoverage=on  Gain=MC_ROLLRATE_I
  Scope : Scope
  Scope1 : Scope
  Scope2 : Scope
  Sum : Sum  Inputs=+++
  Sum1 : Sum  Inputs=|+-
  y : Outport  InitialOutput=0
  wires:
  Integral Gain/1 -> Discrete-Time Integrator/1
  Derivative Gain/1 -> Discrete Derivative/1
  Gain/1 -> Scope/1, Sum/1
  Sum/1 -> y/1
  Discrete Derivative/1 -> Scope2/1, Sum/3
  Discrete-Time Integrator/1 -> Scope1/1, Sum/2
  rollrate_sp/1 -> Sum1/1
  p/1 -> Sum1/2, Gain1/1
  Sum1/1 -> Gain/1, Integral Gain/1
  Gain1/1 -> Derivative Gain/1

== system PosControl_Sim_PID/Control System/Control System/AttitudeControl/PID_yawrate ==
  yawrare_sp : Inport
  r : Inport  Port=2
  Derivative Gain : Gain  DisableCoverage=on  Gain=MC_YAWRATE_D  ParamMin=-100  ParamMax=100  OutMin=-100  OutMax=100
  Discrete Derivative : simulink/Discrete/Discrete Derivative  gainval=1.0  ICPrevScaledInput=0.0  OutMin=[]  OutMax=[]  OutDataType=fixdt(1, 16)  OutScaling=2^-10  DoSatur=off
  Discrete-Time Integrator : DiscreteIntegrator  SampleTime=-1  LimitOutput=on  UpperSaturationLimit=Saturation_I_Y_Max  LowerSaturationLimit=Saturation_I_Y_Min  ICPrevOutput=DiscIntNeverNeededParam  ICPrevScaledInput=DiscIntNeverNeededParam
  Gain : Gain  Gain=MC_YAWRATE_P
  Gain1 : Gain
  Integral Gain : Gain  DisableCoverage=on  Gain=MC_YAWRATE_I
  Sum : Sum  Inputs=+++
  Sum1 : Sum  Inputs=|+-
  y : Outport  InitialOutput=0
  wires:
  Integral Gain/1 -> Discrete-Time Integrator/1
  Derivative Gain/1 -> Discrete Derivative/1
  Gain/1 -> Sum/1
  Sum/1 -> y/1
  Discrete Derivative/1 -> Sum/3
  Discrete-Time Integrator/1 -> Sum/2
  yawrare_sp/1 -> Sum1/1
  r/1 -> Gain1/1, Sum1/2
  Sum1/1 -> Gain/1, Integral Gain/1
  Gain1/1 -> Derivative Gain/1

== system PosControl_Sim_PID/Control System/Control System/position_control/px ==
  ex : Inport
  Gain1 : Gain  Gain=MPC_XY_P
  Saturation3 : Saturate  UpperLimit=MAX_CONTROL_VELOCITY_XY  LowerLimit=-MAX_CONTROL_VELOCITY_XY
  vxd : Outport
  wires:
  ex/1 -> Gain1/1
  Saturation3/1 -> vxd/1
  Gain1/1 -> Saturation3/1

== system PosControl_Sim_PID/Control System/Control System/position_control/py ==
  ey : Inport
  Gain1 : Gain  Gain=MPC_XY_P
  Saturation3 : Saturate  UpperLimit=MAX_CONTROL_VELOCITY_XY  LowerLimit=-MAX_CONTROL_VELOCITY_XY
  vyd : Outport
  wires:
  Gain1/1 -> Saturation3/1
  Saturation3/1 -> vyd/1
  ey/1 -> Gain1/1

== system PosControl_Sim_PID/Control System/Control System/position_control/pz ==
  ez : Inport
  Gain1 : Gain  Gain=MPC_Z_P
  Saturation3 : Saturate  UpperLimit=MAX_CONTROL_VELOCITY_Z  LowerLimit=-MAX_CONTROL_VELOCITY_Z
  vzd : Outport
  wires:
  ez/1 -> Gain1/1
  Saturation3/1 -> vzd/1
  Gain1/1 -> Saturation3/1

== system PosControl_Sim_PID/Control System/Control System/position_control/vx  ==
  vx_d : Inport
  vx : Inport  Port=2
  Derivative Gain : Gain  DisableCoverage=on  Gain=MPC_XY_VEL_D_ACC
  Discrete Derivative : simulink/Discrete/Discrete Derivative  gainval=1.0  ICPrevScaledInput=0.0  OutMin=[]  OutMax=[]  OutDataType=fixdt(1, 16)  OutScaling=2^-10  DoSatur=off
  Discrete-Time Integrator : DiscreteIntegrator  SampleTime=-1  LimitOutput=on  UpperSaturationLimit=Saturation_I_ah  LowerSaturationLimit=-Saturation_I_ah  ICPrevOutput=DiscIntNeverNeededParam  ICPrevScaledInput=DiscIntNeverNeededParam
  Gain : Gain  Gain=MPC_XY_VEL_P_ACC
  Gain1 : Gain  Gain=-1
  Integral Gain : Gain  DisableCoverage=on  Gain=MPC_XY_VEL_I_ACC
  Scope : Scope
  Scope1 : Scope
  Scope2 : Scope
  Sum : Sum  Inputs=+++
  Sum1 : Sum  Inputs=|+-
  y : Outport  InitialOutput=0
  wires:
  Integral Gain/1 -> Discrete-Time Integrator/1
  Derivative Gain/1 -> Discrete Derivative/1
  Gain/1 -> Scope/1, Sum/1
  Sum/1 -> y/1
  Discrete Derivative/1 -> Scope2/1, Sum/3
  Discrete-Time Integrator/1 -> Scope1/1, Sum/2
  vx_d/1 -> Sum1/1
  vx/1 -> Gain1/1, Sum1/2
  Sum1/1 -> Integral Gain/1, Gain/1
  Gain1/1 -> Derivative Gain/1

== system PosControl_Sim_PID/Control System/Control System/position_control/vy  ==
  x : Inport
  Derivative Gain : Gain  DisableCoverage=on  Gain=MPC_XY_VEL_D_ACC
  Discrete Derivative : simulink/Discrete/Discrete Derivative  gainval=1.0  ICPrevScaledInput=0.0  OutMin=-5  OutMax=5  OutDataType=fixdt(1, 16)  OutScaling=2^-10  DoSatur=off
  Discrete-Time Integrator : DiscreteIntegrator  SampleTime=-1  LimitOutput=on  UpperSaturationLimit=Saturation_I_ah  LowerSaturationLimit=-Saturation_I_ah  ICPrevOutput=DiscIntNeverNeededParam  ICPrevScaledInput=DiscIntNeverNeededParam
  Gain : Gain  Gain=MPC_XY_VEL_P_ACC
  Integral Gain : Gain  DisableCoverage=on  Gain=MPC_XY_VEL_I_ACC
  Sum : Sum  Inputs=+++  OutMin=-5  OutMax=5
  y : Outport  InitialOutput=0
  wires:
  x/1 -> Gain/1, Integral Gain/1, Derivative Gain/1
  Integral Gain/1 -> Discrete-Time Integrator/1
  Derivative Gain/1 -> Discrete Derivative/1
  Gain/1 -> Sum/1
  Sum/1 -> y/1
  Discrete Derivative/1 -> Sum/3
  Discrete-Time Integrator/1 -> Sum/2

== system PosControl_Sim_PID/Control System/Control System/position_control/vz  ==
  x : Inport
  Derivative Gain : Gain  DisableCoverage=on  Gain=MPC_Z_VEL_D_ACC
  Discrete Derivative : simulink/Discrete/Discrete Derivative  gainval=1.0  ICPrevScaledInput=0.0  OutMin=[]  OutMax=[]  OutDataType=fixdt(1, 16)  OutScaling=2^-10  DoSatur=off
  Discrete-Time Integrator : DiscreteIntegrator  SampleTime=-1  LimitOutput=on  UpperSaturationLimit=Saturation_I_az  LowerSaturationLimit=-Saturation_I_az  ICPrevOutput=DiscIntNeverNeededParam  ICPrevScaledInput=DiscIntNeverNeededParam
  Gain : Gain  Gain=MPC_Z_VEL_P_ACC
  Integral Gain : Gain  DisableCoverage=on  Gain=MPC_Z_VEL_I_ACC
  Mux : Mux  Inputs=3
  Scope : Scope
  Sum : Sum  Inputs=+++
  y : Outport  InitialOutput=0
  wires:
  Discrete-Time Integrator/1 -> Sum/2
  Discrete Derivative/1 -> Sum/3
  Sum/1 -> y/1
  Gain/1 -> Mux/1, Sum/1
  Derivative Gain/1 -> Mux/3, Discrete Derivative/1
  Integral Gain/1 -> Mux/2, Discrete-Time Integrator/1
  x/1 -> Derivative Gain/1, Integral Gain/1, Gain/1
  Mux/1 -> Scope/1

== system PosControl_Sim_PID/Quadcopter Dynamics/Rigid Model/Rigid-Body Dynamic Model/J*w ==
  p q r : Inport
  J : Inport  Port=2
  J*w : Product  Multiplication=Matrix(*)
  "J*w " : Outport
  wires:
  J*w/1 -> "J*w "/1
  J/1 -> J*w/1
  p q r/1 -> J*w/2

== matlab function PosControl_Sim_PID/Control System/InputConditioning/deadzone1 ==
  data: u input; y output
function y = fcn(u)
%Function description:
%  Control the range of the remote control input from RCMin to RCMax, and
%  set a dead zone with a dead zone size of ±deadZone. The output y is
%  normalized to 0~1.You can get the RC calibration parameters in QGC.
RCMin = 1100;
RCMax = 1900;
RCMid = (RCMin + RCMax)/2;
deadZoneRate = 0.05;
deadZone = deadZoneRate*(RCMax - RCMin);
k = 1/(RCMax - RCMid - deadZone);
% saturation
if(u < RCMin)
    u = RCMin;
elseif(u > RCMax)
    u = RCMax;
end
% dead zone and normalize
 if(u > RCMid + deadZone)
    y = (u-RCMid - deadZone)*k;
 elseif(u < RCMid - deadZone)
     y = (u - RCMid + deadZone)*k;
 else
     y = 0;
 end

 end

== matlab function PosControl_Sim_PID/Control System/InputConditioning/deadzone2 ==
  data: u input; y output
function y = fcn(u)
%Function description:
%  Control the range of the remote control input from RCMin to RCMax, and
%  set a dead zone with a dead zone size of ±deadZone. The output y is
%  normalized to 0~1.You can get the RC calibration parameters in QGC.
RCMin = 1100;
RCMax = 1900;
RCMid = (RCMin + RCMax)/2;
deadZoneRate = 0.05;
deadZone = deadZoneRate*(RCMax - RCMin);
k = 1/(RCMax - RCMid - deadZone);
% saturation
if(u < RCMin)
    u = RCMin;
elseif(u > RCMax)
    u = RCMax;
end
% dead zone and normalize
 if(u > RCMid + deadZone)
    y = (u-RCMid - deadZone)*k;
 elseif(u < RCMid - deadZone)
     y = (u - RCMid + deadZone)*k;
 else
     y = 0;
 end

 end

== matlab function PosControl_Sim_PID/Control System/InputConditioning/deadzone3 ==
  data: u input; y output
function y = fcn(u)
%Function description:
%  Control the range of the remote control input from RCMin to RCMax, and
%  set a dead zone with a dead zone size of ±deadZone. The output y is
%  normalized to 0~1.You can get the RC calibration parameters in QGC.
RCMin = 1100;
RCMax = 1900;
RCMid = (RCMin + RCMax)/2;
deadZoneRate = 0.05;
deadZone = deadZoneRate*(RCMax - RCMin);
k = 1/(RCMax - RCMid - deadZone);
% saturation
if(u < RCMin)
    u = RCMin;
elseif(u > RCMax)
    u = RCMax;
end
% dead zone and normalize
 if(u > RCMid + deadZone)
    y = (u-RCMid - deadZone)*k;
 elseif(u < RCMid - deadZone)
     y = (u - RCMid + deadZone)*k;
 else
     y = 0;
 end

 end

== matlab function PosControl_Sim_PID/Control System/InputConditioning/deadzone4 ==
  data: u input; y output
function y = fcn(u)
%Function description:
%  Control the range of the remote control input from RCMin to RCMax, and
%  set a dead zone with a dead zone size of ±deadZone. The output y is
%  normalized to 0~1.You can get the RC calibration parameters in QGC.
RCMin = 1100;
RCMax = 1900;
RCMid = (RCMin + RCMax)/2;
deadZoneRate = 0.05;
deadZone = deadZoneRate*(RCMax - RCMin);
k = 1/(RCMax - RCMid - deadZone);
% saturation
if(u < RCMin)
    u = RCMin;
elseif(u > RCMax)
    u = RCMax;
end
% dead zone and normalize
 if(u > RCMid + deadZone)
    y = (u-RCMid - deadZone)*k;
 elseif(u < RCMid - deadZone)
     y = (u - RCMid + deadZone)*k;
 else
     y = 0;
 end

 end

== matlab function PosControl_Sim_PID/Control System/Control System/pwm_out1 ==
  data: Roll input; M1 output; Pitch input; Yaw input; Thrust input; M2 output; M3 output; M4 output
function [M1, M2, M3, M4] = motor_mixer(Roll, Pitch, Yaw, Thrust)
%Function description:
%  Control allocation. The quadrotor type is X-configuration,
%  and the airframe is as follows:
%3↓   1↑
 %  \ /
 %  / \
 %2↑   4↓
%Input：
%  Roll, Pitch, Yaw: attitude controller output.
%  Thrust

idle_PWM = 1000;
scale = 1000;

M1 = (Thrust - Roll + Pitch + Yaw) * scale + idle_PWM;
M2 = (Thrust + Roll - Pitch + Yaw) * scale + idle_PWM;
M3 = (Thrust + Roll + Pitch - Yaw) * scale + idle_PWM;
M4 = (Thrust - Roll - Pitch - Yaw) * scale + idle_PWM;
